simulink model "SB13_stateflow_done"  (R2024b)
settings: Solver=FixedStepDiscrete  StartTime=0.0  StopTime=30  FixedStep=0.05  RelTol=1e-3
undefined symbols (not defined in the file or in its folder): DiscIntNeverNeededParam
settings Model: Creator=admin  LastModifiedBy=admin

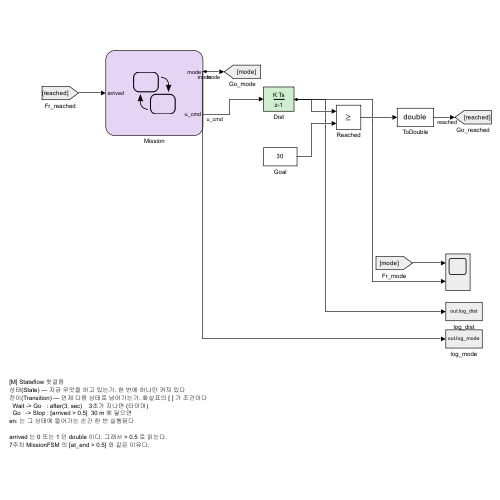
[thumbnail: Simulink's stored preview of the top-level diagram]
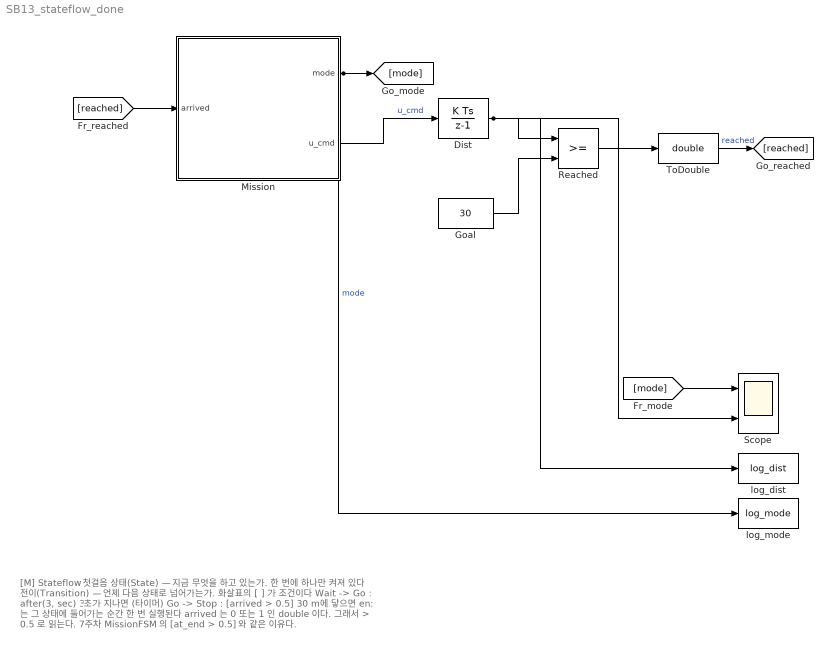
== system SB13_stateflow_done ==
  note: [M] Stateflow 첫걸음
      | 상태(State) — 지금 무엇을 하고 있는가. 한 번에 하나만 켜져 있다
      | 전이(Transition) — 언제 다음 상태로 넘어가는가. 화살표의 [ ] 가 조건이다
      |   Wait -> Go   : after(3, sec)    3초가 지나면 (타이머)
      |   Go   -> Stop : [arrived > 0.5]  30 m 에 닿으면
      | en: 는 그 상태에 들어가는 순간 한 번 실행된다
      |
      | arrived 는 0 또는 1 인 double 이다. 그래서 > 0.5 로 읽는다.
      | 7주차 MissionFSM 의 [at_end > 0.5] 와 같은 이유다.
  Dist : DiscreteIntegrator  SampleTime=0.05  ICPrevOutput=DiscIntNeverNeededParam  ICPrevScaledInput=DiscIntNeverNeededParam
  Goal : Constant  Value=30
  Mission : Stateflow chart  TreatAsAtomicUnit=on
  Reached : RelationalOperator  OutDataTypeStr=boolean  RndMeth=Simplest  InputSameDT=off
  Scope : Scope  NumInputPorts=2
  ToDouble : DataTypeConversion  OutDataTypeStr=double  SaturateOnIntegerOverflow=off  RndMeth=Floor
  log_dist : ToWorkspace  VariableName=log_dist  SaveFormat=Timeseries  SampleTime=0.05
  log_mode : ToWorkspace  VariableName=log_mode  SaveFormat=Timeseries  SampleTime=0.05
  wires:
  Mission/1(mode) -> log_mode/1, [mode]  "mode"
  Mission/2(u_cmd) -> Dist/1  "u_cmd"
  Dist/1 -> Reached/1, log_dist/1, Scope/2
  Goal/1 -> Reached/2
  Reached/1 -> ToDouble/1
  ToDouble/1 -> [reached]  "reached"
  [reached] -> Mission/1(arrived)
  [mode] -> Scope/1

== stateflow chart SB13_stateflow_done/Mission ==
  settings: updateMethod=DISCRETE  sampleTime=0.05
  state Wait
    en: mode = 1; u_cmd = 0;
  state Go
    en: mode = 2; u_cmd = 1.5;
  state Stop
    en: mode = 3; u_cmd = 0;
  (default) -> Wait
  Wait -> Go : after(3, sec)
  Go -> Stop : [arrived > 0.5]
  data: arrived input; mode output; u_cmd output
